simulink model "PInvTemperatureDerate"  (R2024b)
settings: Solver=FixedStepAuto  StartTime=0.0  StopTime=10.0  RelTol=1e-3  EnableMultiTasking=on
settings Model: DataDictionary=Master_Dictionary.sldd  EnableAccessToBaseWorkspace=off  Creator=torni  LastModifiedBy=Will
settings OptimizationCC: DefaultParameterBehavior=Inlined  EnhancedBackFolding=on  PassReuseOutputArgsAs=Individual arguments  ZeroExternalMemoryAtStartup=off  ZeroInternalMemoryAtStartup=off  MaxStackSize=8192  OptimizeBlockOrder=speed  DifferentSizesBufferReuse=on  OptimizationCustomize=off  EfficientTunableParamExpr=on
settings DebuggingCC: ParameterTunabilityLossMsg=error
settings HardwareCC: ProdBitPerPointer=32  ProdBitPerSizeT=32  ProdBitPerPtrDiffT=32  ProdLargestAtomicInteger=Long  ProdLargestAtomicFloat=Double  ProdWordSize=32  ProdLongLongMode=on  ProdHWDeviceType=ARM Compatible->ARM Cortex-M
settings SFSimCC: MATLABDynamicMemAlloc=off
settings RTWCC: Description=Embedded Coder  SystemTargetFile=ert.tlc  HardwareBoard=STM32H7xx Based (Single-core)  TemplateMakefile=ert_default_tmf  Toolchain=GNU Tools for ARM Embedded Processors
settings CodeAppCC: ForceParamTrailComments=on  IgnoreCustomStorageClasses=off  OperatorAnnotations=on  SimulinkDataObjDesc=on  SFDataObjDesc=on  InsertBlockDesc=on
settings ERTTargetCC: TargetLangStandard=C99 (ISO)  CodeReplacementLibrary=ARM Cortex-M  ExtModeTransport=3  ExtModeStaticAlloc=on  ExtModeStaticAllocSize=2048  ExtModeMexFile=ext_xcp  ExtModeIntrfLevel=Level2 - Open

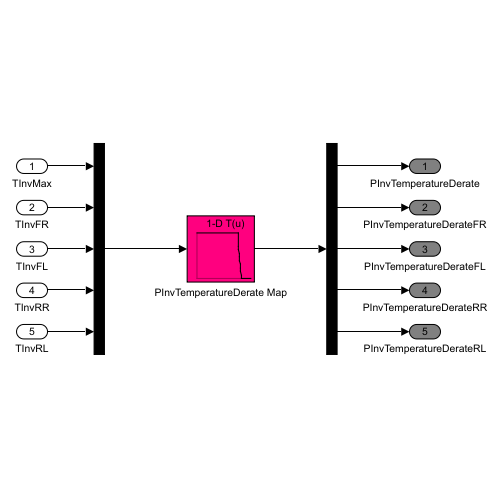
[thumbnail: Simulink's stored preview of the top-level diagram]
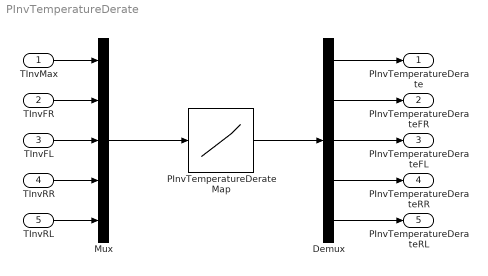
== system PInvTemperatureDerate ==
  "TInvMax " : Inport  OutDataTypeStr=double
  TInvFR : Inport  Port=2  OutDataTypeStr=double
  TInvFL : Inport  Port=3  OutDataTypeStr=double
  TInvRR : Inport  Port=4  OutDataTypeStr=double
  TInvRL : Inport  Port=5  OutDataTypeStr=double
  Demux : Demux  Outputs=5
  Mux : Mux  Inputs=5
  PInvTemperatureDerate Map : Lookup_n-D  NumberOfTableDimensions=1  BreakpointsForDimension1=[0,115,116,117,118,119,120,121,122,123,124,125,150]  Table=[100,100,70.2,62.4,54.6,46.8,39,31.2,23.4,15.6,7.8,0,0]  InternalRulePriority=Speed  RndMeth=Simplest
  PInvTemperatureDerate : Outport  OutDataTypeStr=double  VectorParamsAs1DForOutWhenUnconnected=off
  PInvTemperatureDerateFR : Outport  Port=2  OutDataTypeStr=double  VectorParamsAs1DForOutWhenUnconnected=off
  PInvTemperatureDerateFL : Outport  Port=3  OutDataTypeStr=double  VectorParamsAs1DForOutWhenUnconnected=off
  PInvTemperatureDerateRR : Outport  Port=4  OutDataTypeStr=double  VectorParamsAs1DForOutWhenUnconnected=off
  PInvTemperatureDerateRL : Outport  Port=5  OutDataTypeStr=double  VectorParamsAs1DForOutWhenUnconnected=off
  wires:
  "TInvMax "/1 -> Mux/1
  TInvFR/1 -> Mux/2
  TInvFL/1 -> Mux/3
  TInvRR/1 -> Mux/4
  TInvRL/1 -> Mux/5
  Demux/5 -> PInvTemperatureDerateRL/1
  Demux/4 -> PInvTemperatureDerateRR/1
  Demux/3 -> PInvTemperatureDerateFL/1
  Demux/2 -> PInvTemperatureDerateFR/1
  Demux/1 -> PInvTemperatureDerate/1
  Mux/1 -> PInvTemperatureDerate Map/1
  PInvTemperatureDerate Map/1 -> Demux/1
